simulink model "rispostaCaso2"  (R2023a)
settings: Solver=ode4  StartTime=0.0  StopTime=30  FixedStep=0.001  RelTol=1e-3
model workspace (MAT data in the model file):
  s = tf
  s.IOSize_ = [1 1]
  s.Data_ = ltipack.tfdata
  s.Data_.num = {[1 0]}
  s.Data_.den = {[0 1]}
  s.Data_.Delay.Input = 0
  s.Data_.Delay.Output = 0
  s.Data_.Delay.IO = 0
  s.Data_.Ts = 0
settings Model: Creator=Manuele  LastModifiedBy=Manuele

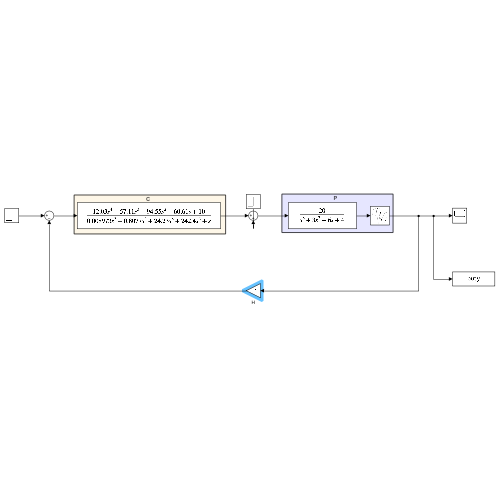
[thumbnail: Simulink's stored preview of the top-level diagram]
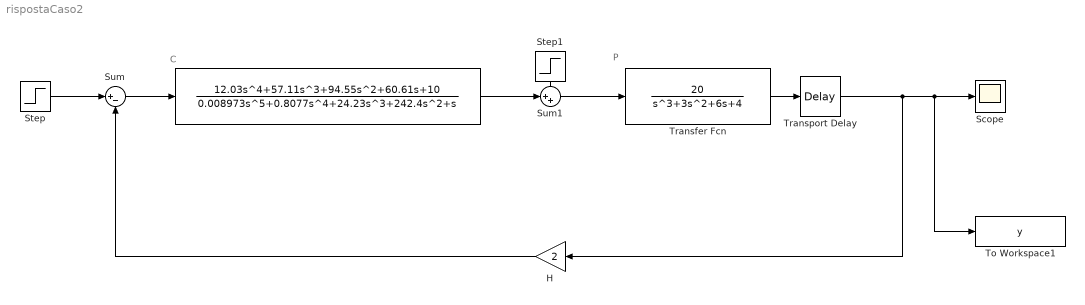
== system rispostaCaso2 ==
  note: C
  note: P
  " " : TransferFcn  Numerator=[12.03 57.11 94.55 60.61 10]  Denominator=[0.008973 0.8077 24.23 242.4 1 0]
  H : Gain  Gain=2
  Scope : Scope
  Step : Step  Time=0  After=0  SampleTime=0
  Step1 : Step  Time=0  Before=3  After=3  SampleTime=0
  Sum : Sum  Inputs=|+-
  Sum1 : Sum  Inputs=|++
  To Workspace1 : ToWorkspace  VariableName=y  SaveFormat=Timeseries  SampleTime=-1
  Transfer Fcn : TransferFcn  Numerator=[20]  Denominator=[1 3 6 4]
  Transport Delay : TransportDelay  DelayTime=0.1
  wires:
  H/1 -> Sum/2
  Sum/1 -> " "/1
  Step/1 -> Sum/1
  " "/1 -> Sum1/1
  Step1/1 -> Sum1/2
  Transfer Fcn/1 -> Transport Delay/1
  Sum1/1 -> Transfer Fcn/1
  Transport Delay/1 -> H/1, To Workspace1/1, Scope/1
